simulink model "foxboro_controller_control101"  (R2024a)
settings: Solver=VariableStepAuto  StartTime=0.0  StopTime=endtime  RelTol=1e-3
undefined symbols (not defined in the file or in its folder): K, umax, umin
libraries: cstblocks x2
settings Model: Creator=barsr  LastModifiedBy=Anthony Rossiter
settings RTWCC: GPUComputeCapability=3.5

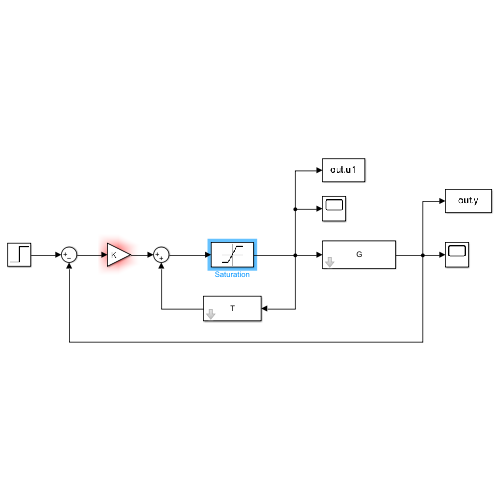
[thumbnail: Simulink's stored preview of the top-level diagram]
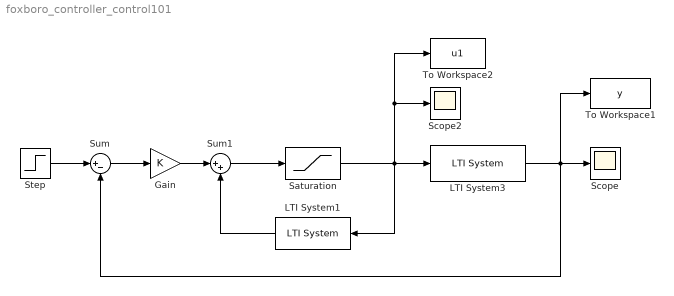
== system foxboro_controller_control101 ==
  Gain : Gain  Gain=K
  LTI System1 : cstblocks/LTI System  sys=T  IC=[]  PadeOrder=0
  LTI System3 : cstblocks/LTI System  sys=G  IC=[]  PadeOrder=0
  Saturation : Saturate  UpperLimit=umax  LowerLimit=umin
  Scope : Scope
  Scope2 : Scope
  Step : Step  Time=0  SampleTime=0
  Sum : Sum  Inputs=|+-
  Sum1 : Sum  Inputs=|++
  To Workspace1 : ToWorkspace  VariableName=y  SaveFormat=Structure With Time  SampleTime=-1
  To Workspace2 : ToWorkspace  VariableName=u1  SaveFormat=Structure With Time  SampleTime=-1
  wires:
  Step/1 -> Sum/1
  Sum/1 -> Gain/1
  Saturation/1 -> LTI System1/1, LTI System3/1, To Workspace2/1, Scope2/1
  LTI System3/1 -> Sum/2, To Workspace1/1, Scope/1
  Gain/1 -> Sum1/1
  LTI System1/1 -> Sum1/2
  Sum1/1 -> Saturation/1
